simulink model "soc_dvbs2_proc"  (R2025b)
settings: Solver=FixedStepDiscrete  StartTime=0.0  StopTime=10  FixedStep=0.001  RelTol=1e-3  EnableMultiTasking=on
model workspace (MAT data in the model file):
  mwTaskManagerKernelLatency = 0
values from neighbouring files (symbols this model uses):
  Rsym = 4e6    (= 4000000)    [soc_dvbs2_init.m]
libraries: prociolib x21
settings Model: DataDictionary=dvbs2hdlReceiverData.sldd  Creator=The MathWorks, Inc.  LastModifiedBy=The MathWorks, Inc.
settings SolverCC: AlgebraicLoopSolver=TrustRegion  PositivePriorityOrder=on  AutoInsertRateTranBlk=on
settings DataIOCC: SaveFormat=StructureWithTime  ReturnWorkspaceOutputs=off
settings OptimizationCC: DefaultParameterBehavior=Inlined  PassReuseOutputArgsAs=Individual arguments  ZeroExternalMemoryAtStartup=off  MaxStackSize=64  EfficientTunableParamExpr=on
settings DebuggingCC: IntegerOverflowMsg=none  ParameterTunabilityLossMsg=error  UnconnectedInputMsg=warning  UnconnectedOutputMsg=warning  UnconnectedLineMsg=warning  SubsystemReferenceDiagnosticForUnitTest=warning  ArithmeticOperatorsInVariantConditions=warning
settings HardwareCC: ProdBitPerLong=64.0  ProdLargestAtomicInteger=LongLong  ProdLargestAtomicFloat=Double  ProdLongLongMode=on  ProdHWDeviceType=ARM Compatible->ARM Cortex-A (64-bit)  HardwareBoardFeatureSet=SoCBlockset
settings ModelReferenceCC: EnableRefExpFcnMdlSchedulingChecks=on  ModelReferenceNumInstancesAllowed=Single
settings SFSimCC: SimUseLocalCustomCode=off
settings RTWCC: SystemTargetFile=ert.tlc  HardwareBoard=Xilinx Zynq UltraScale+ RFSoC ZCU111 Evaluation Kit  TLCOptions="-aInlineSetEventsForThisBaseRateFcn=TLC_FALSE -aSuppressMultiTaskScheduler=TLC_FALSE  -aRateBasedStepFcn=0"  GenCodeOnly=on  TemplateMakefile=ert_default_tmf  GenerateReport=on  RTWUseLocalCustomCode=off  Toolchain=Linaro AArch64 Linux v6.3.1  IncludeHyperlinkInReport=on  LaunchReport=on  CodeExecutionProfiling=on  GenerateTraceInfo=on  GenerateTraceReport=on  GenerateTraceReportSl=on  GenerateTraceReportSf=on  GenerateTraceReportEml=on  GPUComputeCapability=3.5  DLArmComputeVersion=19.05  Description=Embedded Coder
settings CodeAppCC: ForceParamTrailComments=on  IgnoreCustomStorageClasses=off  OperatorAnnotations=on  SimulinkDataObjDesc=on  SFDataObjDesc=on  InsertBlockDesc=on
settings ERTTargetCC: InlinedParameterPlacement=Hierarchical  SupportVariableSizeSignals=on

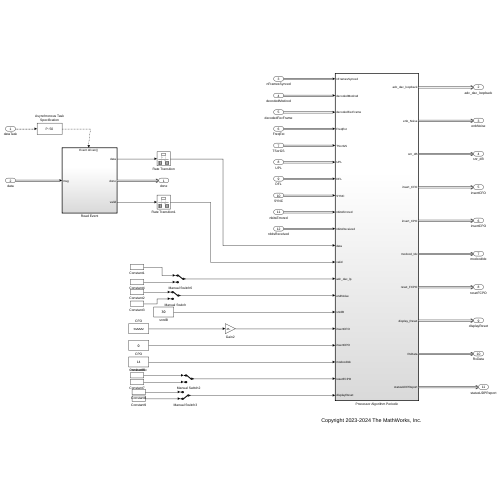
[thumbnail: Simulink's stored preview of the top-level diagram]
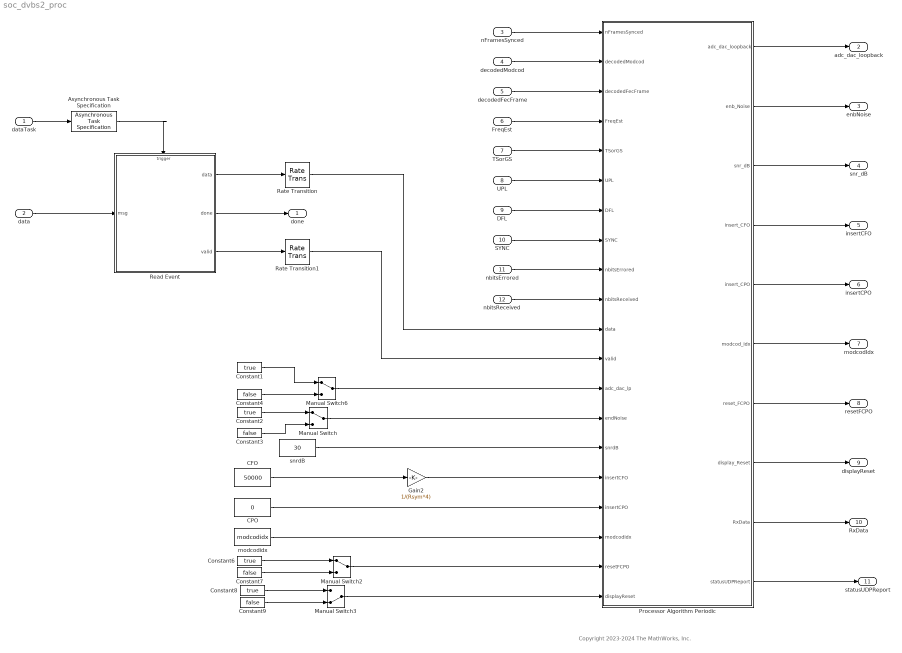
== system soc_dvbs2_proc ==
  note: Copyright 2023-2024 The MathWorks, Inc.
  dataTask : Inport  OutputFunctionCall=on
  data : Inport  OutputPortMessageModes=m  Port=2
  nFramesSynced : Inport  OutputPortMessageModes=m  Port=3
  decodedModcod : Inport  OutputPortMessageModes=m  Port=4
  decodedFecFrame : Inport  OutputPortMessageModes=m  Port=5
  FreqEst : Inport  OutputPortMessageModes=m  Port=6
  TSorGS : Inport  OutputPortMessageModes=m  Port=7
  UPL : Inport  OutputPortMessageModes=m  Port=8
  DFL : Inport  OutputPortMessageModes=m  Port=9
  SYNC : Inport  OutputPortMessageModes=m  Port=10
  nbitsErrored : Inport  OutputPortMessageModes=m  Port=11
  nbitsReceived : Inport  OutputPortMessageModes=m  Port=12
  Asynchronous Task Specification : AsynchronousTaskSpecification  TaskPriority=50
  CFO : Constant  Value=50000  VectorParams1D=off  SampleTime=1e-3
  CPO : Constant  Value=0  OutDataTypeStr=fixdt(1,21,21)  SampleTime=1e-3
  Constant{1..2,6,8} (4 alike) : Constant  Value=true  SampleTime=1e-3
  Constant{3..4,7,9} (4 alike) : Constant  Value=false  SampleTime=1e-3
  Gain2 : Gain  Gain=1/(Rsym*4)  OutDataTypeStr=fixdt(1,21,21)
  Manual Switch : ManualSwitch
  Manual Switch2 : ManualSwitch
  Manual Switch3 : ManualSwitch  CurrentSetting=0
  Manual Switch6 : ManualSwitch
  Processor Algorithm Periodic : Subsystem  TreatAsAtomicUnit=on
  Rate Transition : RateTransition  Deterministic=off  OutPortSampleTime=1e-3
  Rate Transition1 : RateTransition  Deterministic=off  OutPortSampleTime=1e-3
  Read Event : Subsystem
  modcodidx : Constant  Value=modcodidx  OutDataTypeStr=fixdt(0,5,0)  SampleTime=1e-3  mask{modcodvalue=14}
      mask prompts: modcodvalue "MODCOD :"
      mask init:
      | modcodidx = modcodvalue - 1;
      mask TypeOptions modcodvalue: 1 | 2 | 3 | 4 | 5 | 6 | 7 | 8 | 9 | 10 | 12 | 13 | 14 | 15 | 16 | 18 | 19 | 20 | 21 | 22 | 24 | 25 | 26 | 27
      mask Display: disp(get_param(gcb,'modcodvalue'));
  snrdB : Constant  Value=30  OutDataTypeStr=fixdt(1,16,9)  SampleTime=1e-3
  done : Outport  InputPortMessageModes=m
  adc_dac_loopback : Outport  InputPortMessageModes=m  Port=2
  enbNoise : Outport  InputPortMessageModes=m  Port=3
  snr_dB : Outport  InputPortMessageModes=m  Port=4
  insertCFO : Outport  InputPortMessageModes=m  Port=5
  insertCPO : Outport  InputPortMessageModes=m  Port=6
  modcodIdx : Outport  InputPortMessageModes=m  Port=7
  resetFCPO : Outport  InputPortMessageModes=m  Port=8
  displayReset : Outport  InputPortMessageModes=m  Port=9
  RxData : Outport  InputPortMessageModes=m  Port=10
  statusUDPReport : Outport  InputPortMessageModes=m  Port=11
  wires:
  Constant6/1 -> Manual Switch2/1
  Rate Transition1/1 -> Processor Algorithm Periodic/12(valid)
  Manual Switch3/1 -> Processor Algorithm Periodic/20(displayReset)
  Processor Algorithm Periodic/9(RxData) -> RxData/1
  data/1 -> Read Event/1(msg)
  FreqEst/1 -> Processor Algorithm Periodic/4(FreqEst)
  Manual Switch/1 -> Processor Algorithm Periodic/14(endNoise)
  Constant1/1 -> Manual Switch6/1
  Constant7/1 -> Manual Switch2/2
  nbitsErrored/1 -> Processor Algorithm Periodic/9(nbitsErrored)
  Processor Algorithm Periodic/6(modcod_Idx) -> modcodIdx/1
  Processor Algorithm Periodic/8(display_Reset) -> displayReset/1
  nFramesSynced/1 -> Processor Algorithm Periodic/1(nFramesSynced)
  Constant9/1 -> Manual Switch3/2
  Read Event/2(done) -> done/1
  Processor Algorithm Periodic/1(adc_dac_loopback) -> adc_dac_loopback/1
  Read Event/3(valid) -> Rate Transition1/1
  CFO/1 -> Gain2/1
  Constant2/1 -> Manual Switch/1
  Manual Switch2/1 -> Processor Algorithm Periodic/19(resetFCPO)
  UPL/1 -> Processor Algorithm Periodic/6(UPL)
  Processor Algorithm Periodic/10(statusUDPReport) -> statusUDPReport/1
  Processor Algorithm Periodic/4(insert_CFO) -> insertCFO/1
  SYNC/1 -> Processor Algorithm Periodic/8(SYNC)
  Constant4/1 -> Manual Switch6/2
  Processor Algorithm Periodic/3(snr_dB) -> snr_dB/1
  Manual Switch6/1 -> Processor Algorithm Periodic/13(adc_dac_lp)
  Processor Algorithm Periodic/5(insert_CPO) -> insertCPO/1
  modcodidx/1 -> Processor Algorithm Periodic/18(modcodIdx)
  CPO/1 -> Processor Algorithm Periodic/17(insertCPO)
  Gain2/1 -> Processor Algorithm Periodic/16(insertCFO)
  Processor Algorithm Periodic/2(enb_Noise) -> enbNoise/1
  dataTask/1 -> Asynchronous Task Specification/1
  Constant3/1 -> Manual Switch/2
  decodedFecFrame/1 -> Processor Algorithm Periodic/3(decodedFecFrame)
  TSorGS/1 -> Processor Algorithm Periodic/5(TSorGS)
  Rate Transition/1 -> Processor Algorithm Periodic/11(data)
  DFL/1 -> Processor Algorithm Periodic/7(DFL)
  Constant8/1 -> Manual Switch3/1
  Asynchronous Task Specification/1 -> Read Event/Trigger
  decodedModcod/1 -> Processor Algorithm Periodic/2(decodedModcod)
  Processor Algorithm Periodic/7(reset_FCPO) -> resetFCPO/1
  nbitsReceived/1 -> Processor Algorithm Periodic/10(nbitsReceived)
  snrdB/1 -> Processor Algorithm Periodic/15(snrdB)
  Read Event/1(data) -> Rate Transition/1

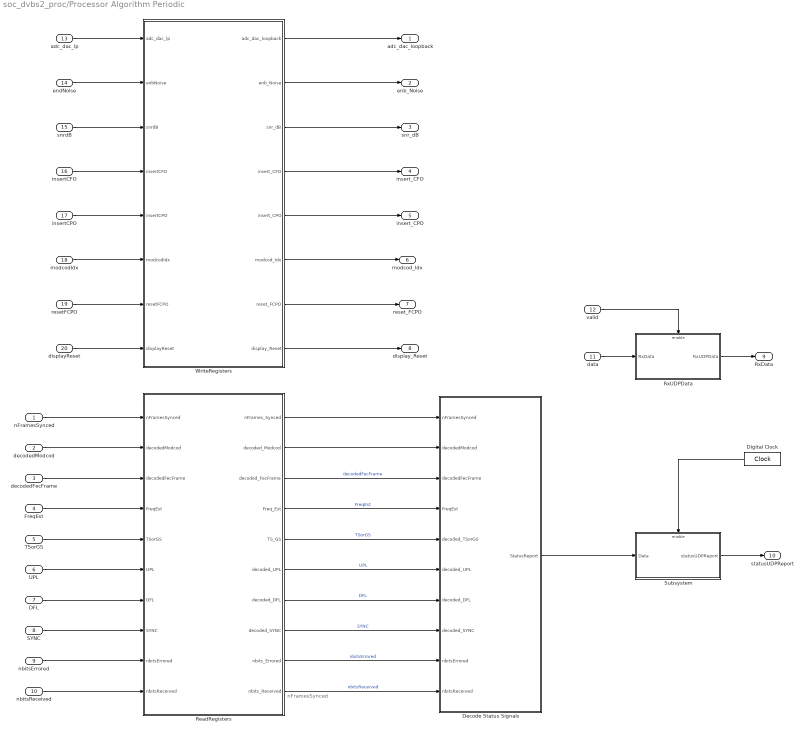
== system soc_dvbs2_proc/Processor Algorithm Periodic ==
  note: nFramesSynced
  nFramesSynced : Inport
  decodedModcod : Inport  Port=2
  decodedFecFrame : Inport  Port=3
  FreqEst : Inport  Port=4
  TSorGS : Inport  Port=5
  UPL : Inport  Port=6
  DFL : Inport  Port=7
  SYNC : Inport  Port=8
  nbitsErrored : Inport  Port=9
  nbitsReceived : Inport  Port=10
  data : Inport  Port=11
  valid : Inport  Port=12
  adc_dac_lp : Inport  Port=13
  endNoise : Inport  Port=14
  snrdB : Inport  Port=15
  insertCFO : Inport  Port=16
  insertCPO : Inport  Port=17
  modcodIdx : Inport  Port=18
  resetFCPO : Inport  Port=19
  displayReset : Inport  Port=20
  Decode Status Signals : Subsystem
  Digital Clock : DigitalClock  SampleTime=1e-3
  ReadRegisters : Subsystem  Priority=10
  RxUDPData : Subsystem
  Subsystem : Subsystem
  WriteRegisters : Subsystem  Priority=1
  adc_dac_loopback : Outport
  enb_Noise : Outport  Port=2
  snr_dB : Outport  Port=3
  insert_CFO : Outport  Port=4
  insert_CPO : Outport  Port=5
  modcod_Idx : Outport  Port=6
  reset_FCPO : Outport  Port=7
  display_Reset : Outport  Port=8
  RxData : Outport  Port=9
  statusUDPReport : Outport  Port=10
  wires:
  WriteRegisters/1(adc_dac_loopback) -> adc_dac_loopback/1
  WriteRegisters/2(enb_Noise) -> enb_Noise/1
  WriteRegisters/7(reset_FCPO) -> reset_FCPO/1
  WriteRegisters/6(modcod_Idx) -> modcod_Idx/1
  WriteRegisters/5(insert_CPO) -> insert_CPO/1
  WriteRegisters/3(snr_dB) -> snr_dB/1
  SYNC/1 -> ReadRegisters/8(SYNC)
  nbitsReceived/1 -> ReadRegisters/10(nbitsReceived)
  decodedFecFrame/1 -> ReadRegisters/3(decodedFecFrame)
  nbitsErrored/1 -> ReadRegisters/9(nbitsErrored)
  FreqEst/1 -> ReadRegisters/4(FreqEst)
  TSorGS/1 -> ReadRegisters/5(TSorGS)
  UPL/1 -> ReadRegisters/6(UPL)
  DFL/1 -> ReadRegisters/7(DFL)
  data/1 -> RxUDPData/1(RxData)
  ReadRegisters/10(nbits_Received) -> Decode Status Signals/10(nbitsReceived)  "nbitsReceived"
  ReadRegisters/9(nbits_Errored) -> Decode Status Signals/9(nbitsErrored)  "nbitsErrored"
  ReadRegisters/8(decoded_SYNC) -> Decode Status Signals/8(decoded_SYNC)  "SYNC"
  ReadRegisters/7(decoded_DFL) -> Decode Status Signals/7(decoded_DFL)  "DFL"
  ReadRegisters/6(decoded_UPL) -> Decode Status Signals/6(decoded_UPL)  "UPL"
  ReadRegisters/5(TS_GS) -> Decode Status Signals/5(decoded_TSorGS)  "TSorGS"
  ReadRegisters/4(Freq_Est) -> Decode Status Signals/4(FreqEst)  "FreqEst"
  ReadRegisters/3(decoded_FecFrame) -> Decode Status Signals/3(decodedFecFrame)  "decodedFecFrame"
  RxUDPData/1(RxUDPData) -> RxData/1
  adc_dac_lp/1 -> WriteRegisters/1(adc_dac_lp)
  displayReset/1 -> WriteRegisters/8(displayReset)
  endNoise/1 -> WriteRegisters/2(enbNoise)
  resetFCPO/1 -> WriteRegisters/7(resetFCPO)
  modcodIdx/1 -> WriteRegisters/6(modcodIdx)
  insertCPO/1 -> WriteRegisters/5(insertCPO)
  snrdB/1 -> WriteRegisters/3(snrdB)
  Decode Status Signals/1(StatusReport) -> Subsystem/1(Data)
  Subsystem/1(statusUDPReport) -> statusUDPReport/1
  valid/1 -> RxUDPData/Enable
  Digital Clock/1 -> Subsystem/Enable
  insertCFO/1 -> WriteRegisters/4(insertCFO)
  WriteRegisters/4(insert_CFO) -> insert_CFO/1
  decodedModcod/1 -> ReadRegisters/2(decodedModcod)
  ReadRegisters/2(decoded_Modcod) -> Decode Status Signals/2(decodedModcod)
  nFramesSynced/1 -> ReadRegisters/1(nFramesSynced)
  ReadRegisters/1(nFrames_Synced) -> Decode Status Signals/1(nFramesSynced)
  WriteRegisters/8(display_Reset) -> display_Reset/1

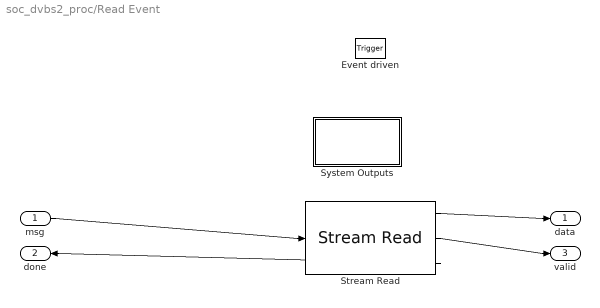
== system soc_dvbs2_proc/Read Event ==
  msg : Inport
  Event driven : TriggerPort  TriggerType=function-call  VariantControl=Variant  PortDimensions=1
  Stream Read : prociolib/Stream Read  DeviceName=mwdvbs2_ip0:s2mm0  OutDataTypeStr=uint32  SamplesPerFrame=RxFrameSize  NumberOfBuffers=4  EnableEvent=on  SampleTime=-1
  System Outputs : Subsystem  mask(System Outputs){ShowInLibBrowser=0}
      mask prompts: ShowInLibBrowser "Simulink:masks:CustCodeMaskParam1_MP"
      settings: CopyFcn=cccopyfcn(gcb)  OpenFcn=ccopenfcn('System Outputs Function')
      mask Help: eval('feval(''rtwprivate'',''rtwhelpview'',''rtw_sys_outputs_block'')');
      mask Display: disp('System\nOutputs');
  data : Outport
  done : Outport  Port=2
  valid : Outport  Port=3
  wires:
  Stream Read/2 -> valid/1
  msg/1 -> Stream Read/1
  Stream Read/3 -> done/1
  Stream Read/1 -> data/1

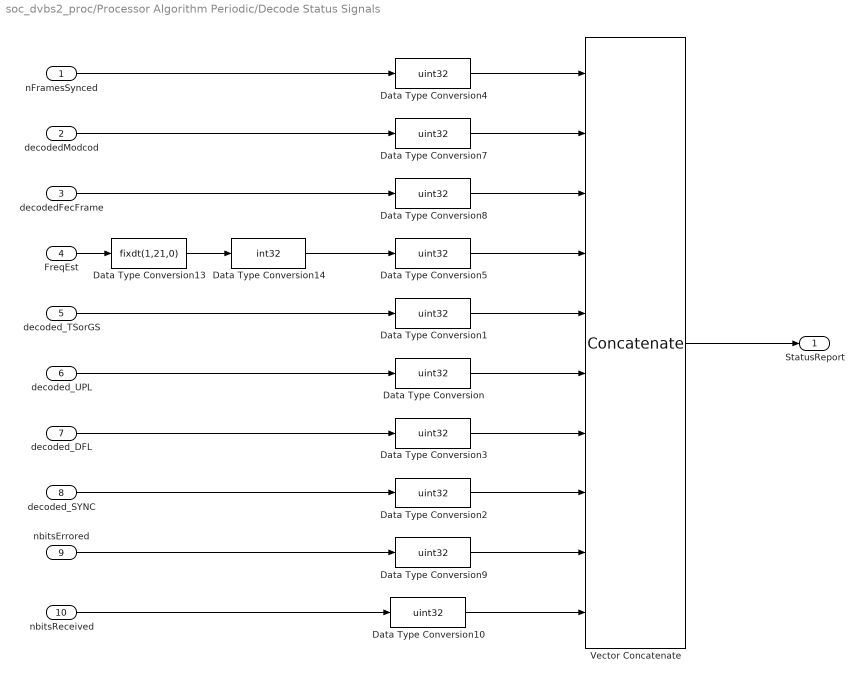
== system soc_dvbs2_proc/Processor Algorithm Periodic/Decode Status Signals ==
  nFramesSynced : Inport
  decodedModcod : Inport  Port=2
  decodedFecFrame : Inport  Port=3
  FreqEst : Inport  Port=4
  decoded_TSorGS : Inport  Port=5
  decoded_UPL : Inport  Port=6
  decoded_DFL : Inport  Port=7
  decoded_SYNC : Inport  Port=8
  nbitsErrored : Inport  Port=9
  nbitsReceived : Inport  Port=10
  Data Type Conversion{,1..5,7..10} (10 alike) : DataTypeConversion  OutDataTypeStr=uint32  SaturateOnIntegerOverflow=off  RndMeth=Floor
  Data Type Conversion13 : DataTypeConversion  OutDataTypeStr=fixdt(1,21,0)  ConvertRealWorld=Stored Integer (SI)  SaturateOnIntegerOverflow=off  RndMeth=Floor
  Data Type Conversion14 : DataTypeConversion  OutDataTypeStr=int32  SaturateOnIntegerOverflow=off  RndMeth=Floor
  Vector Concatenate : Concatenate  NumInputs=10
  StatusReport : Outport
  wires:
  Vector Concatenate/1 -> StatusReport/1
  decoded_DFL/1 -> Data Type Conversion3/1
  decodedFecFrame/1 -> Data Type Conversion8/1
  decoded_TSorGS/1 -> Data Type Conversion1/1
  decoded_UPL/1 -> Data Type Conversion/1
  decoded_SYNC/1 -> Data Type Conversion2/1
  decodedModcod/1 -> Data Type Conversion7/1
  FreqEst/1 -> Data Type Conversion13/1
  nFramesSynced/1 -> Data Type Conversion4/1
  nbitsReceived/1 -> Data Type Conversion10/1
  Data Type Conversion7/1 -> Vector Concatenate/2
  nbitsErrored/1 -> Data Type Conversion9/1
  Data Type Conversion8/1 -> Vector Concatenate/3
  Data Type Conversion4/1 -> Vector Concatenate/1
  Data Type Conversion13/1 -> Data Type Conversion14/1
  Data Type Conversion14/1 -> Data Type Conversion5/1
  Data Type Conversion5/1 -> Vector Concatenate/4
  Data Type Conversion1/1 -> Vector Concatenate/5
  Data Type Conversion/1 -> Vector Concatenate/6
  Data Type Conversion3/1 -> Vector Concatenate/7
  Data Type Conversion2/1 -> Vector Concatenate/8
  Data Type Conversion9/1 -> Vector Concatenate/9
  Data Type Conversion10/1 -> Vector Concatenate/10

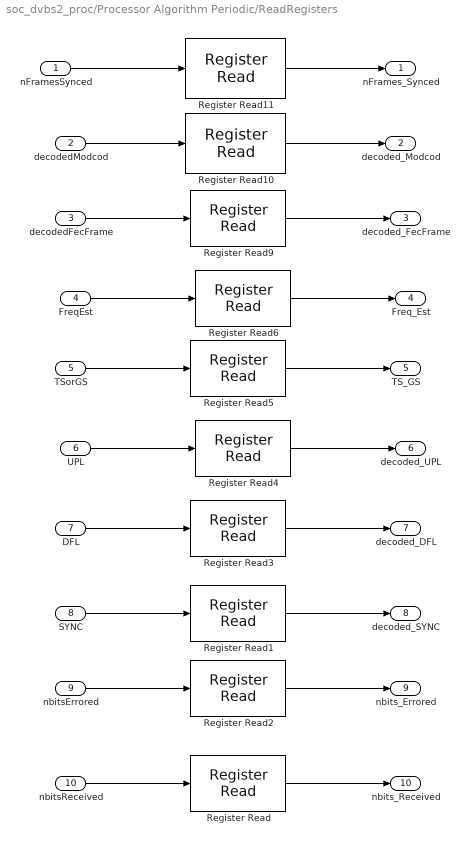
== system soc_dvbs2_proc/Processor Algorithm Periodic/ReadRegisters ==
  nFramesSynced : Inport
  decodedModcod : Inport  Port=2
  decodedFecFrame : Inport  Port=3
  FreqEst : Inport  Port=4
  TSorGS : Inport  Port=5
  UPL : Inport  Port=6
  DFL : Inport  Port=7
  SYNC : Inport  Port=8
  nbitsErrored : Inport  Port=9
  nbitsReceived : Inport  Port=10
  Register Read : prociolib/Register Read  DeviceName=/dev/mwdvbs2_ip0  OffsetAddress=hex2dec('0128')  OutDataTypeStr=uint32  OutputVectorSize=1  SampleTime=-1  Dummy=0
  Register Read1 : prociolib/Register Read  DeviceName=/dev/mwdvbs2_ip0  OffsetAddress=hex2dec('0120')  OutDataTypeStr=uint8  OutputVectorSize=1  SampleTime=-1  Dummy=0
  Register Read10 : prociolib/Register Read  DeviceName=/dev/mwdvbs2_ip0  OffsetAddress=hex2dec('0104')  OutDataTypeStr=fixdt(0,5,0)  OutputVectorSize=1  SampleTime=-1  Dummy=0
  Register Read11 : prociolib/Register Read  DeviceName=/dev/mwdvbs2_ip0  OffsetAddress=hex2dec('0100')  OutDataTypeStr=uint32  OutputVectorSize=1  SampleTime=-1  Dummy=0
  Register Read2 : prociolib/Register Read  DeviceName=/dev/mwdvbs2_ip0  OffsetAddress=hex2dec('0124')  OutDataTypeStr=uint32  OutputVectorSize=1  SampleTime=-1  Dummy=0
  Register Read3 : prociolib/Register Read  DeviceName=/dev/mwdvbs2_ip0  OffsetAddress=hex2dec('011C')  OutDataTypeStr=uint16  OutputVectorSize=1  SampleTime=-1  Dummy=0
  Register Read4 : prociolib/Register Read  DeviceName=/dev/mwdvbs2_ip0  OffsetAddress=hex2dec('0118')  OutDataTypeStr=uint16  OutputVectorSize=1  SampleTime=-1  Dummy=0
  Register Read5 : prociolib/Register Read  DeviceName=/dev/mwdvbs2_ip0  OffsetAddress=hex2dec('0114')  OutDataTypeStr=fixdt(0,2,0)  OutputVectorSize=1  SampleTime=-1  Dummy=0
  Register Read6 : prociolib/Register Read  DeviceName=/dev/mwdvbs2_ip0  OffsetAddress=hex2dec('0110')  OutDataTypeStr=fixdt(1,21,21)  OutputVectorSize=1  SampleTime=-1  Dummy=0
  Register Read9 : prociolib/Register Read  DeviceName=/dev/mwdvbs2_ip0  OffsetAddress=hex2dec('0108')  OutDataTypeStr=fixdt(0,1,0)  OutputVectorSize=1  SampleTime=-1  Dummy=0
  nFrames_Synced : Outport
  decoded_Modcod : Outport  Port=2
  decoded_FecFrame : Outport  Port=3
  Freq_Est : Outport  Port=4
  TS_GS : Outport  Port=5
  decoded_UPL : Outport  Port=6
  decoded_DFL : Outport  Port=7
  decoded_SYNC : Outport  Port=8
  nbits_Errored : Outport  Port=9
  nbits_Received : Outport  Port=10
  wires:
  nbitsReceived/1 -> Register Read/1
  nbitsErrored/1 -> Register Read2/1
  SYNC/1 -> Register Read1/1
  DFL/1 -> Register Read3/1
  UPL/1 -> Register Read4/1
  TSorGS/1 -> Register Read5/1
  FreqEst/1 -> Register Read6/1
  decodedFecFrame/1 -> Register Read9/1
  Register Read/1 -> nbits_Received/1
  Register Read2/1 -> nbits_Errored/1
  Register Read1/1 -> decoded_SYNC/1
  Register Read3/1 -> decoded_DFL/1
  Register Read4/1 -> decoded_UPL/1
  Register Read5/1 -> TS_GS/1
  Register Read6/1 -> Freq_Est/1
  Register Read9/1 -> decoded_FecFrame/1
  decodedModcod/1 -> Register Read10/1
  Register Read10/1 -> decoded_Modcod/1
  nFramesSynced/1 -> Register Read11/1
  Register Read11/1 -> nFrames_Synced/1

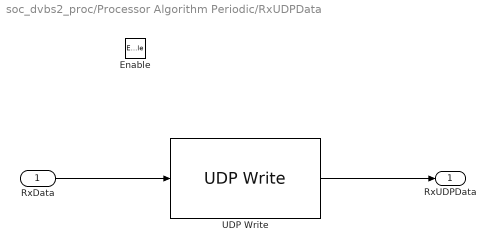
== system soc_dvbs2_proc/Processor Algorithm Periodic/RxUDPData ==
  RxData : Inport
  Enable : EnablePort
  UDP Write : prociolib/UDP Write  RemoteAddress=255.255.255.255  RemotePort=25000  LocalPort=-1  ByteOrder=LittleEndian  OutputStatus=off  hoistedMaskSrc=Variant/CODEGEN/UDP Write
  RxUDPData : Outport  VectorParamsAs1DForOutWhenUnconnected=off
  wires:
  UDP Write/1 -> RxUDPData/1
  RxData/1 -> UDP Write/1

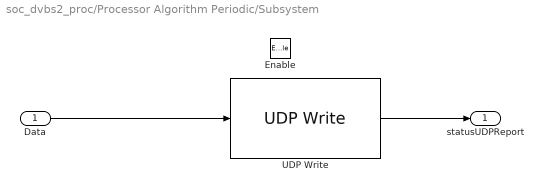
== system soc_dvbs2_proc/Processor Algorithm Periodic/Subsystem ==
  Data : Inport
  Enable : EnablePort
  UDP Write : prociolib/UDP Write  RemoteAddress=255.255.255.255  RemotePort=25001  LocalPort=-1  ByteOrder=LittleEndian  OutputStatus=off  hoistedMaskSrc=Variant/CODEGEN/UDP Write
  statusUDPReport : Outport
  wires:
  UDP Write/1 -> statusUDPReport/1
  Data/1 -> UDP Write/1

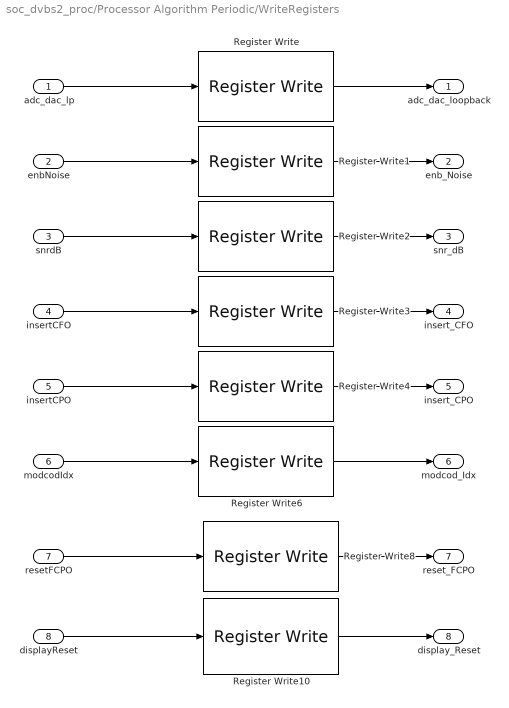
== system soc_dvbs2_proc/Processor Algorithm Periodic/WriteRegisters ==
  adc_dac_lp : Inport
  enbNoise : Inport  Port=2
  snrdB : Inport  Port=3
  insertCFO : Inport  Port=4
  insertCPO : Inport  Port=5
  modcodIdx : Inport  Port=6
  resetFCPO : Inport  Port=7
  displayReset : Inport  Port=8
  Register Write : prociolib/Register Write  OutputSink=To output port  TunableParamName=A  RegisterName=RegA  DeviceName=/dev/mwdvbs2_ip0  OffsetAddress=hex2dec('012C')  Dummy=0
  Register Write1 : prociolib/Register Write  OutputSink=To output port  TunableParamName=A  RegisterName=RegA  DeviceName=/dev/mwdvbs2_ip0  OffsetAddress=hex2dec('0130')  Dummy=0
  Register Write10 : prociolib/Register Write  OutputSink=To output port  TunableParamName=A  RegisterName=RegA  DeviceName=/dev/mwdvbs2_ip0  OffsetAddress=hex2dec('0148')  Dummy=0
  Register Write2 : prociolib/Register Write  OutputSink=To output port  TunableParamName=A  RegisterName=RegA  DeviceName=/dev/mwdvbs2_ip0  OffsetAddress=hex2dec('0134')  Dummy=0
  Register Write3 : prociolib/Register Write  OutputSink=To output port  TunableParamName=A  RegisterName=RegA  DeviceName=/dev/mwdvbs2_ip0  OffsetAddress=hex2dec('0138')  Dummy=0
  Register Write4 : prociolib/Register Write  OutputSink=To output port  TunableParamName=A  RegisterName=RegA  DeviceName=/dev/mwdvbs2_ip0  OffsetAddress=hex2dec('013C')  Dummy=0
  Register Write6 : prociolib/Register Write  OutputSink=To output port  TunableParamName=A  RegisterName=RegA  DeviceName=/dev/mwdvbs2_ip0  OffsetAddress=hex2dec('0140')  Dummy=0
  Register Write8 : prociolib/Register Write  OutputSink=To output port  TunableParamName=A  RegisterName=RegA  DeviceName=/dev/mwdvbs2_ip0  OffsetAddress=hex2dec('0144')  Dummy=0
  adc_dac_loopback : Outport
  enb_Noise : Outport  Port=2
  snr_dB : Outport  Port=3
  insert_CFO : Outport  Port=4
  insert_CPO : Outport  Port=5
  modcod_Idx : Outport  Port=6
  reset_FCPO : Outport  Port=7
  display_Reset : Outport  Port=8
  wires:
  adc_dac_lp/1 -> Register Write/1
  Register Write/1 -> adc_dac_loopback/1
  enbNoise/1 -> Register Write1/1
  Register Write1/1 -> enb_Noise/1
  snrdB/1 -> Register Write2/1
  Register Write2/1 -> snr_dB/1
  insertCFO/1 -> Register Write3/1
  Register Write3/1 -> insert_CFO/1
  insertCPO/1 -> Register Write4/1
  Register Write4/1 -> insert_CPO/1
  modcodIdx/1 -> Register Write6/1
  Register Write6/1 -> modcod_Idx/1
  resetFCPO/1 -> Register Write8/1
  Register Write8/1 -> reset_FCPO/1
  displayReset/1 -> Register Write10/1
  Register Write10/1 -> display_Reset/1

== system soc_dvbs2_proc/Read Event/System Outputs ==
